simulink model "sim04"  (R2020a)
settings: Solver=VariableStepAuto  StartTime=0.0  StopTime=25  RelTol=1e-3
values from neighbouring files (symbols this model uses):
  a = 4    [lab04.m]
  b = 13    [lab04.m]
  c = 3    [lab04.m]
  du = 0    [lab04.m]
  k = 2    [lab04.m]
  u0 = 1    [lab04.m]
  x0 = 0    [lab04.m]
  x10 = 0    [lab04.m]
settings Model: Creator=jakub  LastModifiedBy=jakub

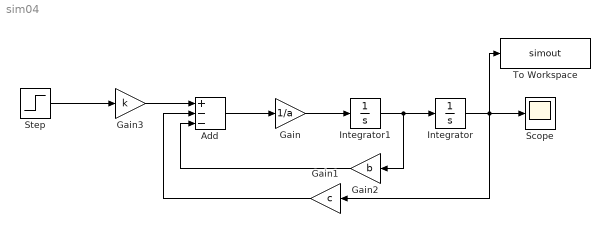
== system sim04 ==
  Add : Sum  Inputs=+--
  Gain : Gain  Gain=1/a
  Gain1 : Gain  Gain=c
  Gain2 : Gain  Gain=b
  Gain3 : Gain  Gain=k
  Integrator : Integrator  InitialCondition=x0
  Integrator1 : Integrator  InitialCondition=x10
  Scope : Scope
  Step : Step  Time=0  Before=u0  After=u0+du  SampleTime=0
  To Workspace : ToWorkspace  VariableName=simout  SampleTime=-1
  wires:
  Integrator1/1 -> Gain2/1, Integrator/1
  Gain/1 -> Integrator1/1
  Add/1 -> Gain/1
  Integrator/1 -> Gain1/1, To Workspace/1, Scope/1
  Gain2/1 -> Add/3
  Gain1/1 -> Add/2
  Step/1 -> Gain3/1
  Gain3/1 -> Add/1
